simulink model "MPC_design"  (R2019b)
settings: Solver=FixedStepAuto  StartTime=0.0  StopTime=10.0  FixedStep=0.025  RelTol=1e-3
values from neighbouring files (symbols this model uses):
  A1 = [-4.40211640212 20.8695652174 167280.42328 290539.68254 -0.830687830688 -5.1867826087 -10253.968254 54825.3968254 0 0 -1.26886956522 2.93843478261 ... (16 elements, 4x4)]    [MPC_object_design_params_twooutputs.mat]    (also in model_generate.m = [a11 a12 a13 a14)
  B1 = [1.60846560847 15.8608695652 -61121.6931217 -106158.730159 0 0 38000 0 0 0.000347826086957 -1.05739130435 2.44869565217 ... (16 elements, 4x4)]    [MPC_object_design_params_twooutputs.mat]    (also in model_generate.m = [b11 b12 b13 b14)
  C1 = [1 0 0 0 0 1 0 0 0 0 1 0 ... (16 elements, 4x4)]    [MPC_object_design_params_twooutputs.mat]    (also in model_generate.m = eye(4))
  D1 = [0 0 0 0 0 0 0 0 0 0 0 0 ... (16 elements, 4x4)]    [MPC_object_design_params_twooutputs.mat]    (also in model_generate.m = zeros(4,4))
undefined symbols (not defined in the file or in its folder): C2, D2
libraries: mpclib x2
settings Model: Creator=shouv  LastModifiedBy=shouv

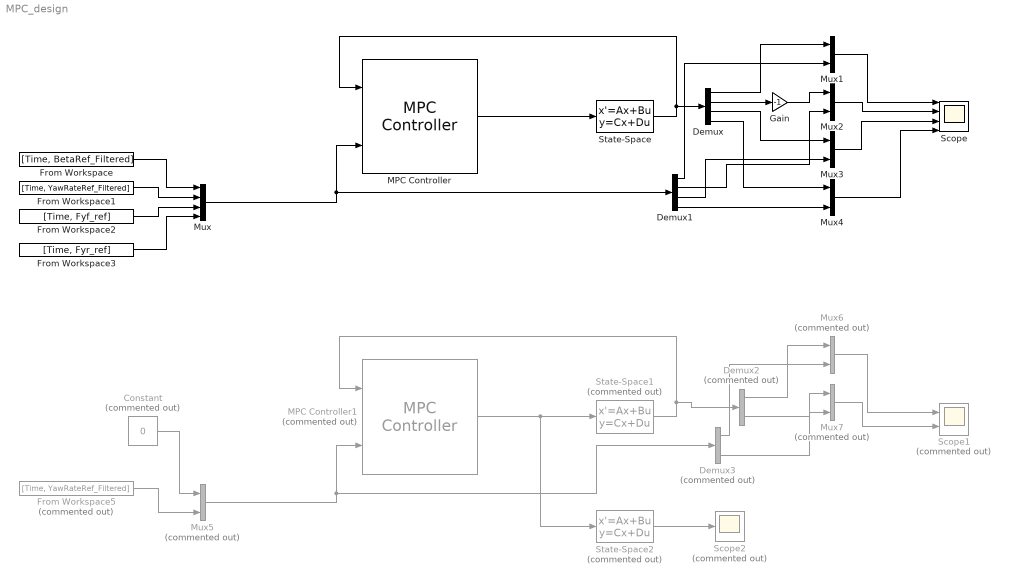
== system MPC_design ==
  Constant : Constant  Commented=on  Value=0
  Demux : Demux
  Demux1 : Demux
  Demux2 : Demux  Commented=on  Outputs=2
  Demux3 : Demux  Commented=on  Outputs=2
  From Workspace : FromWorkspace  VariableName=[Time, BetaRef_Filtered]  SampleTime=0
  From Workspace1 : FromWorkspace  VariableName=[Time, YawRateRef_Filtered]  SampleTime=0
  From Workspace2 : FromWorkspace  VariableName=[Time, Fyf_ref]  SampleTime=0
  From Workspace3 : FromWorkspace  VariableName=[Time, Fyr_ref]  SampleTime=0
  From Workspace5 : FromWorkspace  Commented=on  VariableName=[Time, YawRateRef_Filtered]  SampleTime=0
  Gain : Gain  Gain=-1
  MPC Controller : mpclib/MPC Controller  SCDEnableBlockLinearizationSpecification=on  mpcobj=mpc1  is_multiple=0  enable_value=0  return_u0=off  updateMPCinCallerWorkspace=on  md_inport=off  mv_inport=off  uref_inport=off  return_cost=off  return_mvseq=off  return_qpstatus=off  return_xseq=off  return_state=off  return_ovseq=off  state_inport=off  umin_inport=off  umax_inport=off  ymin_inport=off  ymax_inport=off  cc_inport=off  ywt_inport=off  uwt_inport=off  duwt_inport=off  rhoeps_inport=off  pm_inport=off  MaximumP=10  HorizonChoice=FixedHorizon  n_ts=0.1  n_p=15  n_mv=4  n_md=0  n_ud=0  n_mo=4  n_uo=0  BlockDataType=double  SampleTimeInherited=off  switch_inport=off
  MPC Controller1 : mpclib/MPC Controller  Commented=on  SCDEnableBlockLinearizationSpecification=on  mpcobj=mpc1  is_multiple=0  enable_value=0  return_u0=off  updateMPCinCallerWorkspace=on  md_inport=off  mv_inport=off  uref_inport=off  return_cost=off  return_mvseq=off  return_qpstatus=off  return_xseq=off  return_state=off  return_ovseq=off  state_inport=off  umin_inport=off  umax_inport=off  ymin_inport=off  ymax_inport=off  cc_inport=off  ywt_inport=off  uwt_inport=off  duwt_inport=off  rhoeps_inport=off  pm_inport=off  MaximumP=10  HorizonChoice=FixedHorizon  n_ts=0.1  n_p=10  n_mv=4  n_md=0  n_ud=0  n_mo=2  n_uo=0  BlockDataType=double  SampleTimeInherited=off  switch_inport=off
  Mux : Mux
  Mux{1..4} (4 alike) : Mux  Inputs=2
  Mux5 : Mux  Commented=on  Inputs=2
  Mux6 : Mux  Commented=on  Inputs=2
  Mux7 : Mux  Commented=on  Inputs=2
  Scope : Scope  NumInputPorts=4
  Scope1 : Scope  Commented=on  NumInputPorts=2
  Scope2 : Scope  Commented=on
  State-Space : StateSpace  A=A1  B=B1  C=C1  D=D1  InitialCondition=0
  State-Space1 : StateSpace  Commented=on  A=A1  B=B1  C=C1  D=D1  InitialCondition=0
  State-Space2 : StateSpace  Commented=on  A=A1  B=B1  C=C2  D=D2  InitialCondition=0
  wires:
  MPC Controller/1 -> State-Space/1
  State-Space/1 -> MPC Controller/1, Demux/1
  Mux/1 -> Demux1/1, MPC Controller/2
  From Workspace1/1 -> Mux/2
  From Workspace2/1 -> Mux/3
  From Workspace/1 -> Mux/1
  From Workspace3/1 -> Mux/4
  Demux/1 -> Mux1/1
  Demux/2 -> Gain/1
  Demux/3 -> Mux3/1
  Demux/4 -> Mux4/1
  Demux1/1 -> Mux1/2
  Demux1/2 -> Mux2/2
  Demux1/3 -> Mux3/2
  Demux1/4 -> Mux4/2
  Mux2/1 -> Scope/2
  Mux3/1 -> Scope/3
  Mux1/1 -> Scope/1
  Mux4/1 -> Scope/4
  State-Space1/1 -> Demux2/1, MPC Controller1/1
  MPC Controller1/1 -> State-Space2/1, State-Space1/1
  Mux6/1 -> Scope1/1
  Demux3/1 -> Mux6/2
  Demux3/2 -> Mux7/2
  Mux7/1 -> Scope1/2
  From Workspace5/1 -> Mux5/2
  Demux2/1 -> Mux6/1
  Demux2/2 -> Mux7/1
  Mux5/1 -> Demux3/1, MPC Controller1/2
  Gain/1 -> Mux2/1
  State-Space2/1 -> Scope2/1
  Constant/1 -> Mux5/1
